simulink model "ContinuousDiffSwerveModuleSimulation"  (R2022a)
settings: Solver=VariableStepAuto  StartTime=0.0  StopTime=100  RelTol=1e-3
values from neighbouring files (symbols this model uses):
  A = [0   1.0000        0        0 ... (first row only)    [invgui.m]    (also in pitchgui.m = [-0.313       56.7    0; rscale.m = a)
  B = [0; 1.8182; 0; 4.5455]    [invgui.m]    (also in pitchgui.m = [0.232; rscale.m = b)
  C = [1 0 0 0]    [invgui.m]    (also in pitchgui.m = [0 0 1]; rscale.m = c)
  D = [0]    [invgui.m]    (also in pitchgui.m; rscale.m = d)
undefined symbols (not defined in the file or in its folder): Kff, lqr_K
settings Model: Creator=benjaminwarwick  LastModifiedBy=woz4t

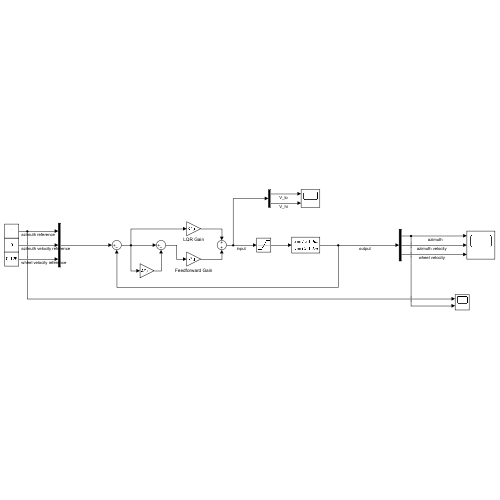
[thumbnail: Simulink's stored preview of the top-level diagram]
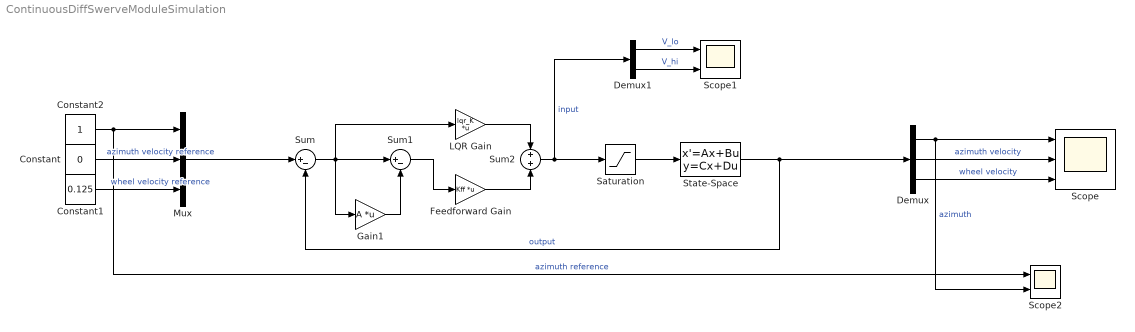
== system ContinuousDiffSwerveModuleSimulation ==
  Constant : Constant  Value=0
  Constant1 : Constant  Value=0.125
  Constant2 : Constant
  Demux : Demux  Outputs=3
  Demux1 : Demux  Outputs=2
  Feedforward Gain : Gain  Gain=Kff  Multiplication=Matrix(K*u)
  Gain1 : Gain  Gain=A  Multiplication=Matrix(K*u)
  LQR Gain : Gain  Gain=lqr_K  Multiplication=Matrix(K*u)
  Mux : Mux  Inputs=3
  Saturation : Saturate  UpperLimit=12  LowerLimit=-12
  Scope : Scope  NumInputPorts=3
  Scope1 : Scope  NumInputPorts=2
  Scope2 : Scope  NumInputPorts=2
  State-Space : StateSpace  A=A  B=B  C=C  D=D  InitialCondition=0  ContinuousStateAttributes={'azimuth', 'azimuth_vel', 'wheel_vel'}
  Sum : Sum  Inputs=|+-
  Sum1 : Sum  Inputs=|+-
  Sum2 : Sum
  wires:
  State-Space/1 -> Sum/2, Demux/1  "output"
  Demux/1 -> Scope2/2, Scope/1  "azimuth"
  Demux/2 -> Scope/2  "azimuth velocity"
  Demux/3 -> Scope/3  "wheel velocity"
  Constant/1 -> Mux/2  "azimuth velocity reference"
  Constant1/1 -> Mux/3  "wheel velocity reference"
  Mux/1 -> Sum/1
  Sum2/1 -> Demux1/1, Saturation/1  "input"
  Sum/1 -> LQR Gain/1, Sum1/1, Gain1/1
  Gain1/1 -> Sum1/2
  Feedforward Gain/1 -> Sum2/2
  LQR Gain/1 -> Sum2/1
  Demux1/1 -> Scope1/1  "V_lo"
  Demux1/2 -> Scope1/2  "V_hi"
  Constant2/1 -> Scope2/1, Mux/1  "azimuth reference"
  Saturation/1 -> State-Space/1
  Sum1/1 -> Feedforward Gain/1
